simulink library "SimscapeCustomComponents_lib"  (R2025b)
settings: Solver=VariableStepAuto  StartTime=0.0  StopTime=10.0  RelTol=1e-3
undefined symbols (not defined in the file or in its folder): base, baseVdc, capacity, DiscIntNeverNeededParam, ee_sli_rtmsupport, filterInductance, freqeuncy, frequency, gcbh, gflInverter, gfmInverter, iMaxPU, Inertia, initialSOC, plantRating, solar, Ts, ups, Vac, windSystem, windTurbine
libraries: fl_lib x397, nesl_utility x171, eeGeneralControl x85, ee_lib x82, simulink x72, datacenter_lib x68, eeTransforms x38, slpidlib x24, buildingEnergy_lib x20, SimscapeFluids_lib x17, eeSinusoidalMeasurementV2 x8, eePwmGenerator x8
(part 19 of 24)

== system SimscapeCustomComponents_lib/Microgrid and Renewables/Control/BESS/Grid Forming Control/VoltageCurrentControl/Controller/Voltage control ==
  e : Inport
  resetBlackStart : Inport  Port=2
  Discrete-Time Integrator : DiscreteIntegrator  IntegratorMethod=Integration: Backward Euler  ExternalReset=level  SampleTime=voltControlTs  LimitOutput=on  UpperSaturationLimit=VdMaxCt  LowerSaturationLimit=VdMinCt  ICPrevOutput=DiscIntNeverNeededParam  ICPrevScaledInput=DiscIntNeverNeededParam
  Ki : Gain  Gain=VdIGain
  Kp : Gain  Gain=vdPGain
  Limit : Saturate  UpperLimit=VdMaxCt  LowerLimit=VdMinCt
  Scope : Scope  NumInputPorts=2
      settings: ActiveDisplayYMinimum=-2.29888  ActiveDisplayYMaximum=11.36654  DataLoggingVariableName=ScopeData7
  Scope1 : Scope
      settings: ActiveDisplayYMinimum=-0.22989  ActiveDisplayYMaximum=1.13665  DataLoggingVariableName=ScopeData8
  Sum7 : Sum  Inputs=|++
  u : Outport  VectorParamsAs1DForOutWhenUnconnected=off
  wires:
  Discrete-Time Integrator/1 -> Sum7/2, Scope/2
  Kp/1 -> Sum7/1, Scope/1
  Limit/1 -> u/1
  Ki/1 -> Discrete-Time Integrator/1
  Sum7/1 -> Limit/1
  e/1 -> Kp/1, Ki/1, Scope1/1
  resetBlackStart/1 -> Discrete-Time Integrator/2

== system SimscapeCustomComponents_lib/Microgrid and Renewables/Control/BESS/Grid Forming Control/VoltageCurrentControl/Controller/Voltage control1 ==
  e : Inport
  resetBlackStart : Inport  Port=2
  Discrete-Time Integrator : DiscreteIntegrator  IntegratorMethod=Integration: Backward Euler  ExternalReset=level  SampleTime=voltControlTs  LimitOutput=on  UpperSaturationLimit=VqMaxCt  LowerSaturationLimit=VqMinCt  ICPrevOutput=DiscIntNeverNeededParam  ICPrevScaledInput=DiscIntNeverNeededParam
  Ki : Gain  Gain=VqIGain
  Kp : Gain  Gain=VqPGain
  Limit : Saturate  UpperLimit=VqMaxCt  LowerLimit=VqMinCt
  Sum7 : Sum  Inputs=|++
  u : Outport  VectorParamsAs1DForOutWhenUnconnected=off
  wires:
  Discrete-Time Integrator/1 -> Sum7/2
  Sum7/1 -> Limit/1
  e/1 -> Ki/1, Kp/1
  Kp/1 -> Sum7/1
  Ki/1 -> Discrete-Time Integrator/1
  Limit/1 -> u/1
  resetBlackStart/1 -> Discrete-Time Integrator/2

== system SimscapeCustomComponents_lib/Microgrid and Renewables/Control/BESS/Grid Forming Control/VoltageCurrentControl/Controller/d-axis current control ==
  e : Inport
  resetBlackStart : Inport  Port=2
  Discrete-Time Integrator : DiscreteIntegrator  IntegratorMethod=Integration: Backward Euler  ExternalReset=level  SampleTime=currentControlTs  LimitOutput=on  UpperSaturationLimit=4  LowerSaturationLimit=-4  ICPrevOutput=DiscIntNeverNeededParam  ICPrevScaledInput=DiscIntNeverNeededParam
  Ki : Gain  Gain=IdIGain
  Kp : Gain  Gain=IdPGain
  Limit : Saturate  UpperLimit=4  LowerLimit=-4
  Sum7 : Sum  Inputs=|++
  u : Outport  VectorParamsAs1DForOutWhenUnconnected=off
  wires:
  Discrete-Time Integrator/1 -> Sum7/2
  Sum7/1 -> Limit/1
  e/1 -> Ki/1, Kp/1
  Kp/1 -> Sum7/1
  Limit/1 -> u/1
  Ki/1 -> Discrete-Time Integrator/1
  resetBlackStart/1 -> Discrete-Time Integrator/2

== system SimscapeCustomComponents_lib/Microgrid and Renewables/Control/BESS/Grid Forming Control/VoltageCurrentControl/Controller/q-axis current control ==
  e : Inport
  resetBlackStart : Inport  Port=2
  Discrete-Time Integrator : DiscreteIntegrator  IntegratorMethod=Integration: Backward Euler  ExternalReset=level  SampleTime=currentControlTs  LimitOutput=on  UpperSaturationLimit=3  LowerSaturationLimit=-3  ICPrevOutput=DiscIntNeverNeededParam  ICPrevScaledInput=DiscIntNeverNeededParam
  Ki : Gain  Gain=IqIGain
  Kp : Gain  Gain=IqPGain
  Limit : Saturate  UpperLimit=3  LowerLimit=-3
  Sum7 : Sum  Inputs=|++
  u : Outport  VectorParamsAs1DForOutWhenUnconnected=off
  wires:
  Ki/1 -> Discrete-Time Integrator/1
  Kp/1 -> Sum7/1
  e/1 -> Kp/1, Ki/1
  Sum7/1 -> Limit/1
  Limit/1 -> u/1
  Discrete-Time Integrator/1 -> Sum7/2
  resetBlackStart/1 -> Discrete-Time Integrator/2

== system SimscapeCustomComponents_lib/Microgrid and Renewables/Control/Renewables/Power Reference Controller/Power Reference Controller/Reference Current/Current limits ==
  Imax : Inport
  iqref : Inport  Port=2
  idref : Inport  Port=3
  Constant8 : Constant  Value=0
  Constant9 : Constant  Value=0
  Scope : Scope
      settings: ActiveDisplayYMinimum=-0.15  ActiveDisplayYMaximum=1.35  DataLoggingVariableName=ScopeData3
  Scope1 : Scope
      settings: ActiveDisplayYMinimum=-0.08298  ActiveDisplayYMaximum=0.74678  DataLoggingVariableName=ScopeData4
  Sqrt : Sqrt
  Sqrt1 : Sqrt
  Square{1..4} (4 alike) : Math  Operator=square
  Step2 : Step  Time=0.01  SampleTime=Ts
  Step3 : Step  Time=0.01  SampleTime=Ts
  Sum6 : Sum  Inputs=|+-
  Sum9 : Sum  Inputs=|+-
  Switch1 : Switch  Threshold=.01  SaturateOnIntegerOverflow=off  InputSameDT=off
  Switch2 : Switch  Threshold=.01  SaturateOnIntegerOverflow=off  InputSameDT=off
  iubq : Outport
  iubd : Outport  Port=2
  wires:
  Sum9/1 -> Switch2/1
  Step3/1 -> Switch2/2
  Step2/1 -> Switch1/2
  Switch2/1 -> Sqrt1/1
  Square1/1 -> Sum6/1
  Switch1/1 -> Sqrt/1
  iqref/1 -> Square2/1
  Square3/1 -> Sum9/1
  Sum6/1 -> Switch1/1
  Square2/1 -> Sum6/2
  Constant8/1 -> Switch1/3
  Square4/1 -> Sum9/2
  Constant9/1 -> Switch2/3
  Sqrt/1 -> Scope/1, iubd/1
  Imax/1 -> Square3/1, Square1/1
  Sqrt1/1 -> Scope1/1, iubq/1
  idref/1 -> Square4/1

== system SimscapeCustomComponents_lib/Microgrid and Renewables/Control/Renewables/Power Reference Controller/Power Reference Controller/Reference Current/Refernce id generation ==
  V_mag : Inport
  ubid : Inport  Port=2
  PRef : Inport  Port=3
  Divide : Product  Inputs=/*
  Gain6 : Gain  Gain=-1
  P/Q Priority : Switch  Criteria=u2 ~= 0  SaturateOnIntegerOverflow=off  InputSameDT=off
  Priority Mode : Constant  Value=P-2
  Saturation Dynamic2 : simulink/Discontinuities/Saturation Dynamic  OutMin=[]  OutMax=[]  OutDataTypeStr=Inherit: Same as second input  OutDataType=fixdt(1, 16)  OutScaling=2^-10  DoSatur=off
  Saturation1 : Saturate  UpperLimit=Imax  LowerLimit=-Imax
  Scope : Scope
      settings: ActiveDisplayYMinimum=0.99583  ActiveDisplayYMaximum=1.02853
  Scope1 : Scope
      settings: ActiveDisplayYMinimum=-0.12499  ActiveDisplayYMaximum=1.12489  DataLoggingVariableName=ScopeData2
  ubid1 : InportShadow  Port=2
  id_ref : Outport
  wires:
  PRef/1 -> Divide/2
  ubid/1 -> Saturation Dynamic2/1
  Gain6/1 -> Saturation Dynamic2/3
  Saturation Dynamic2/1 -> Scope1/1, P/Q Priority/3
  Priority Mode/1 -> P/Q Priority/2
  Saturation1/1 -> P/Q Priority/1
  ubid1/1 -> Gain6/1
  P/Q Priority/1 -> Scope/1, id_ref/1
  V_mag/1 -> Divide/1
  Divide/1 -> Saturation Dynamic2/2, Saturation1/1

== system SimscapeCustomComponents_lib/Microgrid and Renewables/Control/Renewables/Power Reference Controller/Power Reference Controller/Reference Current/Refernce iq generation ==
  ubiq : Inport
  V_mag : Inport  Port=2
  LVRT_iq : Inport  Port=3
  Q_ref : Inport  Port=4
  Divide1 : Product  Inputs=*/
  Gain : Gain  Gain=-1
  Gain1 : Gain  Gain=-1
  Gain7 : Gain  Gain=-1
  LVRT Priority : Switch  Threshold=.9  SaturateOnIntegerOverflow=off  InputSameDT=off
  P/Q Priority : Switch  Criteria=u2 ~= 0  SaturateOnIntegerOverflow=off  InputSameDT=off
  Priority Mode : Constant  Value=P-2
  Saturation Dynamic : simulink/Discontinuities/Saturation Dynamic  OutMin=[]  OutMax=[]  OutDataTypeStr=Inherit: Same as second input  OutDataType=fixdt(1, 16)  OutScaling=2^-10  DoSatur=off
  Saturation2 : Saturate  UpperLimit=1  LowerLimit=-1
  Saturation3 : Saturate  UpperLimit=Imax  LowerLimit=-Imax
  Scope : Scope  NumInputPorts=3
      settings: ActiveDisplayYMinimum=-0.025  ActiveDisplayYMaximum=0.22499  DataLoggingVariableName=ScopeData10
  ubiq1 : InportShadow
  iq_ref : Outport
  wires:
  LVRT Priority/1 -> Gain/1
  P/Q Priority/1 -> LVRT Priority/1, Scope/1
  Gain1/1 -> LVRT Priority/3
  ubiq/1 -> Saturation Dynamic/1
  Saturation2/1 -> Gain1/1
  Saturation3/1 -> P/Q Priority/3
  Priority Mode/1 -> P/Q Priority/2
  Divide1/1 -> Saturation3/1, Saturation Dynamic/2
  Saturation Dynamic/1 -> P/Q Priority/1
  Gain7/1 -> Saturation Dynamic/3
  LVRT_iq/1 -> Saturation2/1
  ubiq1/1 -> Gain7/1
  Q_ref/1 -> Divide1/1
  V_mag/1 -> LVRT Priority/2, Divide1/2
  Gain/1 -> iq_ref/1

== system SimscapeCustomComponents_lib/Microgrid and Renewables/Control/Renewables/Solar PV Controller/DC voltage controller & current reference/If Action Subsystem/Subsystem ==
  V mag : Inport
  iq ub : Inport  Port=2
  Q ref : Inport  Port=3
  Constant : Constant  Value=1e-3
  Data Type Conversion Inherited : simulink/Signal Attributes/Data Type Conversion Inherited  ConvertRealWorld=Real World Value  DoSatur=off
  Divide2 : Product  Inputs=*/
  Gain3 : Gain  Gain=-1
  Saturation Dynamic2 : simulink/Discontinuities/Saturation Dynamic  OutMin=[]  OutMax=[]  OutDataTypeStr=Inherit: Same as second input  OutDataType=fixdt(1, 16)  OutScaling=2^-10  DoSatur=off
  Switch : Switch  Criteria=u2 ~= 0  SaturateOnIntegerOverflow=off  InputSameDT=off
  iq ub1 : InportShadow  Port=2
  iqref : Outport
  wires:
  iq ub1/1 -> Gain3/1
  Divide2/1 -> Saturation Dynamic2/2
  Q ref/1 -> Divide2/1
  Gain3/1 -> Saturation Dynamic2/3
  iq ub/1 -> Saturation Dynamic2/1
  Saturation Dynamic2/1 -> iqref/1
  V mag/1 -> Data Type Conversion Inherited/1, Switch/2, Switch/1
  Switch/1 -> Divide2/2
  Constant/1 -> Data Type Conversion Inherited/2
  Data Type Conversion Inherited/1 -> Switch/3

== system SimscapeCustomComponents_lib/Microgrid and Renewables/Control/Renewables/Solar PV Controller/DC voltage controller & current reference/If Action Subsystem/Subsystem1 ==
  Vmag : Inport
  P pv : Inport  Port=2
  vdc : Inport  Port=3
  vdc ref : Inport  Port=4
  id ub : Inport  Port=5
  Constant : Constant  Value=1e-3
  Constant4 : Constant  Value=0
  Data Type Conversion Inherited : simulink/Signal Attributes/Data Type Conversion Inherited  ConvertRealWorld=Real World Value  DoSatur=off
  Divide : Product  Inputs=/*
  Gain4 : Gain  Gain=1/(mVAbase)
  Saturation Dynamic1 : simulink/Discontinuities/Saturation Dynamic  OutMin=[]  OutMax=[]  OutDataTypeStr=Inherit: Same as second input  OutDataType=fixdt(1, 16)  OutScaling=2^-10  DoSatur=off
  Scope : Scope  NumInputPorts=2
      settings: ActiveDisplayYMinimum=-55957.97767  ActiveDisplayYMaximum=503630.2665
  Sum : Sum  Inputs=|++
  Switch : Switch  Criteria=u2 ~= 0  SaturateOnIntegerOverflow=off  InputSameDT=off
  V_dc_Controller1 : Subsystem
  idref : Outport
  wires:
  Constant4/1 -> Saturation Dynamic1/3
  P pv/1 -> Gain4/1
  V_dc_Controller1/1(Out1) -> Sum/2
  Sum/1 -> Saturation Dynamic1/2
  vdc ref/1 -> V_dc_Controller1/2(vdc ref), Scope/2
  id ub/1 -> Saturation Dynamic1/1
  Gain4/1 -> Divide/2
  Divide/1 -> Sum/1
  Saturation Dynamic1/1 -> idref/1
  vdc/1 -> V_dc_Controller1/1(vdc), Scope/1
  Vmag/1 -> Data Type Conversion Inherited/1, Switch/2, Switch/1
  Switch/1 -> Divide/1
  Constant/1 -> Data Type Conversion Inherited/2
  Data Type Conversion Inherited/1 -> Switch/3

== system SimscapeCustomComponents_lib/Microgrid and Renewables/Control/Renewables/Solar PV Controller/DC voltage controller & current reference/Subsystem1/V_dc_Controller1 ==
  vdc : Inport
  vdc ref : Inport  Port=2
  Gain : Gain  Gain=1/VdcBase
  PID Controller : slpidlib/PID Controller  Controller=PID  Form=Parallel  TimeDomain=Discrete-time  UseExternalTs=off  SampleTime=-1  IntegratorMethod=Forward Euler  FilterMethod=Forward Euler  ControllerParametersSource=internal  P=Kpv  I=Kiv  UseKiTs=off  D=Kdv  UseExternalDerivativeSource=off  N=100  UseFilter=on  TunerSelectOption=Transfer Function Based (PID Tuner App)  ZeroCross=off  InitialConditionSource=internal  InitialConditionForIntegrator=0  InitialConditionForFilter=0  DifferentiatorICPrevScaledInput=0  ExternalReset=none  TrackingMode=off  Kt=1  LimitOutput=off  SatLimitsSource=internal  UpperSaturationLimit=iMax  LowerSaturationLimit=0  LinearizeAsGain=on  AntiWindupMode=clamping  Kb=1  LimitIntegrator=off  UpperIntegratorSaturationLimit=inf  LowerIntegratorSaturationLimit=-inf  POutMin=[]  POutMax=[]  IOutMin=[]  IOutMax=[]  DOutMin=[]  DOutMax=[]  NOutMin=[]  NOutMax=[]  SumOutMin=[]  SumOutMax=[]  SaturationOutMin=[]  SaturationOutMax=[]  PParamMin=[]  PParamMax=[]  IParamMin=[]  IParamMax=[]  DParamMin=[]  DParamMax=[]  NParamMin=[]  NParamMax=[]  KbParamMin=[]  KbParamMax=[]  KtParamMin=[]  KtParamMax=[]  KbOutMin=[]  KbOutMax=[]  KtOutMin=[]  KtOutMax=[]  IntegratorOutMin=[]  IntegratorOutMax=[]  FilterOutMin=[]  FilterOutMax=[]  SumI1OutMin=[]  SumI1OutMax=[]  SumI2OutMin=[]  SumI2OutMax=[]  SumI3OutMin=[]  SumI3OutMax=[]  SumI4OutMin=[]  SumI4OutMax=[]  SumDOutMin=[]  SumDOutMax=[]  DifferentiatorOutMin=[]  DifferentiatorOutMax=[]  FilterDiffOutCoefMin=[]  FilterDiffOutCoefMax=[]  ReciprocalOutMin=[]  ReciprocalOutMax=[]  SumDenOutMin=[]  SumDenOutMax=[]  SumNumOutMin=[]  SumNumOutMax=[]  DivideOutMin=[]  DivideOutMax=[]  UdiffTsProdOutMin=[]  UdiffTsProdOutMax=[]  NTsProdOutMin=[]  NTsProdOutMax=[]  UintegralTsProdOutMin=[]  UintegralTsProdOutMax=[]  UngainTsProdOutMin=[]  UngainTsProdOutMax=[]  ClampingZeroOutDataTypeStr=Inherit: Inherit via back propagation  ClampingZeroOutMin=[]  ClampingZeroOutMax=[]  FilterDenConstantOutDataTypeStr=Inherit: Inherit via back propagation  FilterDenConstantOutMin=[]  FilterDenConstantOutMax=[]  PCopyOutDataTypeStr=Inherit: Inherit via back propagation  PCopyOutMin=[]  PCopyOutMax=[]  NCopyOutDataTypeStr=Inherit: Inherit via back propagation  NCopyOutMin=[]  NCopyOutMax=[]  IntegratorContinuousStateAttributes=''  IntegratorStateMustResolveToSignalObject=off  IntegratorRTWStateStorageClass=Auto  FilterContinuousStateAttributes=''  FilterStateMustResolveToSignalObject=off  FilterRTWStateStorageClass=Auto  ParallelPVariant=InternalParameters  IdealPVariant=Disabled  IVariant=InternalParameters  DVariant=InternalParameters  IntegratorVariant=Discrete  SatVariant=Disabled  AWVariant=Passthrough  PCopyVariant=Disabled  TRVariant=Disabled  FdbkBlocksVariant=Forward  IdealPFdbkVariant=Disabled  SatFdbkVariant=Disabled  DerivativeFilterVariant=ForwardEulerFilter  NVariant=InternalParameters  NCopyVariant=Disabled  FilterICVariant=InternalICsFilter  IntegratorICVariant=InternalICs  ExternalResetVariant=Disabled  TRSumVariant=Passthrough  SumFdbkVariant=Disabled  SumVariant=Sum_PID  TsampFilterVariant=InternalTs  TsampNgainVariant=Passthrough  TsampIntegralVariant=Disabled_SignalSpec  ExternalSaturationOutDataTypeStr=Inherit: Same as second input  DerivativeSourceVariant=ErrorSignal  PreIntVariant=InternalPreInt
  Sum : Sum  Inputs=|+-
  Out1 : Outport
  wires:
  vdc/1 -> Sum/1
  vdc ref/1 -> Sum/2
  PID Controller/1 -> Out1/1
  Gain/1 -> PID Controller/1
  Sum/1 -> Gain/1

== system SimscapeCustomComponents_lib/Microgrid and Renewables/Control/Renewables/Wind Controller/Machine Converter Control/Power Controller/Derating Control ==
  Enable : EnablePort  StatesWhenEnabling=reset
  Constant : Constant  Value=windTurbine.turbineRatedPower
  MW to W : Gain  Gain=1e6
  activePowerDemand : Outport
  wires:
  MW to W/1 -> activePowerDemand/1
  Constant/1 -> MW to W/1

== system SimscapeCustomComponents_lib/Microgrid and Renewables/Control/Renewables/Wind Controller/Machine Converter Control/Power Controller/Limiter Function Power Demand ==
  activePowerDemandMPPT : Inport
  activePowerDemandDerating : Inport  Port=2
  Merge : Merge
  activePowerDemand : Outport
  wires:
  activePowerDemandMPPT/1 -> Merge/1
  activePowerDemandDerating/1 -> Merge/2
  Merge/1 -> activePowerDemand/1

== system SimscapeCustomComponents_lib/Microgrid and Renewables/Control/Renewables/Wind Controller/Machine Converter Control/Power Controller/MPPT Control ==
  windSpeed : Inport
  Enable : EnablePort  StatesWhenEnabling=reset
  MW to W : Gain  Gain=1e6
  mpptActivePowerDemand : Lookup_n-D  NumberOfTableDimensions=1  BreakpointsForDimension1=mpptWindSpeed  Table=mpptPower  InternalRulePriority=Speed  RndMeth=Simplest
  activePowerDemand : Outport
  wires:
  mpptActivePowerDemand/1 -> MW to W/1
  windSpeed/1 -> mpptActivePowerDemand/1
  MW to W/1 -> activePowerDemand/1

== system SimscapeCustomComponents_lib/Microgrid and Renewables/Control/Renewables/Wind Controller/Wind Grid-side Converter Controller/Current_controller/PI ==
  Input : Inport
  Discrete-Time Integrator : DiscreteIntegrator  gainval=Kdii_g  SampleTime=Ts  ICPrevOutput=DiscIntNeverNeededParam  ICPrevScaledInput=DiscIntNeverNeededParam
  Gain1 : Gain  Gain=Kdpi_g
  Sum1 : Sum  Inputs=|++
  Unit Delay : UnitDelay  SampleTime=Ts
  Out2 : Outport
  wires:
  Discrete-Time Integrator/1 -> Sum1/1
  Sum1/1 -> Out2/1
  Unit Delay/1 -> Sum1/2
  Gain1/1 -> Unit Delay/1
  Input/1 -> Gain1/1, Discrete-Time Integrator/1

== system SimscapeCustomComponents_lib/Microgrid and Renewables/Control/Renewables/Wind Controller/Wind Grid-side Converter Controller/Current_controller/PI1 ==
  Input : Inport
  Discrete-Time Integrator : DiscreteIntegrator  gainval=Kqii_g  SampleTime=Ts  ICPrevOutput=DiscIntNeverNeededParam  ICPrevScaledInput=DiscIntNeverNeededParam
  Gain1 : Gain  Gain=Kqpi_g
  Sum1 : Sum  Inputs=|++
  Unit Delay : UnitDelay  SampleTime=Ts
  Out2 : Outport
  wires:
  Discrete-Time Integrator/1 -> Sum1/1
  Sum1/1 -> Out2/1
  Unit Delay/1 -> Sum1/2
  Gain1/1 -> Unit Delay/1
  Input/1 -> Gain1/1, Discrete-Time Integrator/1

== system SimscapeCustomComponents_lib/Microgrid and Renewables/Control/Renewables/Wind Controller/Wind Grid-side Converter Controller/DC voltage controller & current reference/Current limits ==
  Imax : Inport
  iqref : Inport  Port=2
  idref : Inport  Port=3
  Constant8 : Constant  Value=0
  Constant9 : Constant  Value=0
  Sqrt : Sqrt
  Sqrt1 : Sqrt
  Square{1..4} (4 alike) : Math  Operator=square
  Step2 : Step  Time=0.01  SampleTime=Ts
  Step3 : Step  Time=0.01  SampleTime=Ts
  Sum6 : Sum  Inputs=|+-
  Sum9 : Sum  Inputs=|+-
  Switch1 : Switch  Threshold=.01  SaturateOnIntegerOverflow=off  InputSameDT=off
  Switch2 : Switch  Threshold=.01  SaturateOnIntegerOverflow=off  InputSameDT=off
  iubq : Outport
  iubd : Outport  Port=2
  wires:
  Sum9/1 -> Switch2/1
  Step3/1 -> Switch2/2
  Step2/1 -> Switch1/2
  Switch2/1 -> Sqrt1/1
  Square1/1 -> Sum6/1
  Switch1/1 -> Sqrt/1
  iqref/1 -> Square2/1
  Square3/1 -> Sum9/1
  Sum6/1 -> Switch1/1
  Square2/1 -> Sum6/2
  Constant8/1 -> Switch1/3
  Square4/1 -> Sum9/2
  Constant9/1 -> Switch2/3
  Sqrt/1 -> iubd/1
  Imax/1 -> Square3/1, Square1/1
  Sqrt1/1 -> iubq/1
  idref/1 -> Square4/1

== system SimscapeCustomComponents_lib/Microgrid and Renewables/Control/Renewables/Wind Controller/Wind Grid-side Converter Controller/DC voltage controller & current reference/Subsystem ==
  V_mag : Inport
  iq_ub : Inport  Port=2
  lvrt.iq : Inport  Port=3
  Q_ref : Inport  Port=4
  Divide2 : Product  Inputs=*/
  Gain3 : Gain  Gain=-1
  Saturation Dynamic2 : simulink/Discontinuities/Saturation Dynamic  OutMin=[]  OutMax=[]  OutDataTypeStr=Inherit: Same as second input  OutDataType=fixdt(1, 16)  OutScaling=2^-10  DoSatur=off
  Switch6 : Switch  Threshold=.9  SaturateOnIntegerOverflow=off  InputSameDT=off
  iq_ub1 : InportShadow  Port=2
  Out1 : Outport
  wires:
  V_mag/1 -> Switch6/2, Divide2/2
  iq_ub1/1 -> Gain3/1
  Divide2/1 -> Saturation Dynamic2/2
  Q_ref/1 -> Divide2/1
  Gain3/1 -> Saturation Dynamic2/3
  iq_ub/1 -> Saturation Dynamic2/1
  Saturation Dynamic2/1 -> Switch6/1
  Switch6/1 -> Out1/1
  lvrt.iq/1 -> Switch6/3

== system SimscapeCustomComponents_lib/Microgrid and Renewables/Control/Renewables/Wind Controller/Wind Grid-side Converter Controller/DC voltage controller & current reference/Subsystem1 ==
  Wind_Mpp_vdc : Inport
  Wind_vdc : Inport  Port=2
  id_ub : Inport  Port=3
  Constant4 : Constant  Value=0
  Saturation Dynamic1 : simulink/Discontinuities/Saturation Dynamic  OutMin=[]  OutMax=[]  OutDataTypeStr=Inherit: Same as second input  OutDataType=fixdt(1, 16)  OutScaling=2^-10  DoSatur=off
  V_dc_Controller1 : Subsystem
  Out1 : Outport
  wires:
  Constant4/1 -> Saturation Dynamic1/3
  V_dc_Controller1/1(Out1) -> Saturation Dynamic1/2
  Wind_vdc/1 -> V_dc_Controller1/2(In2)
  id_ub/1 -> Saturation Dynamic1/1
  Saturation Dynamic1/1 -> Out1/1
  Wind_Mpp_vdc/1 -> V_dc_Controller1/1(Wind_plant1)

== system SimscapeCustomComponents_lib/Microgrid and Renewables/Sources/Solar Plant Integrated/Detailed/PV Plant & Controller/Controller/MPPT ==
  Qref : Inport
  ipv (A) : Inport  Port=2
  vdc (V) : Inport  Port=3
  Vabc : Inport  Port=4
  Iabc : Inport  Port=5
  Action Port : ActionPort
  Solar PV Controller : Subsystem  LoadFcn=ee_sli_rtmsupport( 'loadfcn', gcbh );  mask(Solar PV Controller (Three-Phase)){L=filterInductance, frequency=frequency, iMax=iMaxPU, zBase=Vac^2/(plantRating*1000), mVAbase=plantRating*1000, VdcBase=baseVoltageDC, sampleTime=-1, Choice=Perturb and observe (P&O), Vdc=1100, delV=3, tSettling=1e-3, Kppll=1e-4, Kipll=0.02, initialPhase=0, Kpv=0.1, Kiv=1, Kdv=0, Kpicd=0.01, Kiicd=0.1, Kdicd=0, Kpicq=0.01, Kiicq=0.1, Kdicq=0}
      mask prompts: L "physmod:ee:library:comments:control:eeRenewablesControl:ACFilterInductanceH_MP"; frequency "physmod:ee:library:comments:control:eeRenewablesControl:SystemFrequencyHz_MP"; iMax "physmod:ee:library:comments:control:eeRenewablesControl:InverterCurrentLimitpu_MP"; zBase "physmod:ee:library:comments:control:eeRenewablesControl:BaseImpedanceACSideOhm_MP"; mVAbase "physmod:ee:library:comments:control:eeRenewablesControl:BaseMVA_MP"; VdcBase "physmod:ee:library:comments:control:eeRenewablesControl:DCBusBaseVoltageV_MP"; sampleTime "physmod:ee:library:comments:control:eeRenewablesControl:SampleTime1ForInherited_MP"; Choice "physmod:ee:library:comments:control:eeRenewablesControl:Algorithm_MP"; Vdc "physmod:ee:library:comments:control:eeRenewablesControl:InitialVoltageForMPPTV_MP"; delV "physmod:ee:library:comments:control:eeRenewablesControl:VoltageStepOfMPPTV_MP"; tSettling "physmod:ee:library:comments:control:eeRenewablesControl:SettlingTimeOfMPPTs_MP"; Kppll "physmod:ee:library:comments:control:eeRenewablesControl:ProportionalGain_MP"; Kipll "physmod:ee:library:comments:control:eeRenewablesControl:IntegralGain_MP"; initialPhase "physmod:ee:library:comments:control:eeRenewablesControl:InitialPhaseAngle_MP"; Kpv "physmod:ee:library:comments:control:eeRenewablesControl:ProportionalGain_MP"; Kiv "physmod:ee:library:comments:control:eeRenewablesControl:IntegralGain_MP"; Kdv "physmod:ee:library:comments:control:eeRenewablesControl:DerivativeGain_MP"; Kpicd "physmod:ee:library:comments:control:eeRenewablesControl:DaxisProportionalGain_MP"; Kiicd "physmod:ee:library:comments:control:eeRenewablesControl:DaxisIntegralGain_MP"; Kdicd "physmod:ee:library:comments:control:eeRenewablesControl:DaxisDerivativeGain_MP"; Kpicq "physmod:ee:library:comments:control:eeRenewablesControl:QaxisProportionalGain_MP"; Kiicq "physmod:ee:library:comments:control:eeRenewablesControl:QaxisIntegralGain_MP"; Kdicq "physmod:ee:library:comments:control:eeRenewablesControl:QaxisDerivativeGain_MP"
      mask help: physmod:ee:library:comments:control:eeRenewablesControl:PVGridFollowingController_MD
      mask init: same as SimscapeCustomComponents_lib/Microgrid and Renewables/Control/Renewables/Solar PV Controller
      settings: CopyFcn=ee_sli_rtmsupport( 'copyfcn', gcbh );  DeleteFcn=ee_sli_rtmsupport( 'deletefcn', gcbh );  ModelCloseFcn=ee_sli_rtmsupport( 'modelclosefcn', gcbh );  PostSaveFcn=ee_sli_rtmsupport( 'postsavefcn', gcbh );  PreCopyFcn=ee_sli_rtmsupport( 'precopyfcn', gcbh );  OpenFcn=ee_sli_rtmsupport( 'openfcn', gcbh );  CloseFcn=ee_sli_rtmsupport( 'closefcn', gcbh );  PreDeleteFcn=ee_sli_rtmsupport( 'predeletefcn', gcbh );
      mask Help: web(nesl_help(gcbh))
      mask TypeOptions sampleTime: Current_controller/SystemSampleTime | DC voltage controller & current reference/SystemSampleTime
      mask TypeOptions Choice: Variant Subsystem/LabelModeActiveChoice
      mask DialogControl Container4 Prompt: physmod:ee:library:comments:control:eeRenewablesControl:General_Tab
      mask DialogControl L Prompt: AC filter inductance (H)
      mask DialogControl frequency Prompt: System frequency (Hz)
      mask DialogControl iMax Prompt: Inverter current limit (pu)
      mask DialogControl zBase Prompt: Base impedance on AC side (Ohm)
      mask DialogControl mVAbase Prompt: Base power on AC side (V*A)
      mask DialogControl VdcBase Prompt: DC bus base voltage (V)
      mask DialogControl sampleTime Prompt: Sample time (-1 for inherited)
      mask DialogControl Container5 Prompt: physmod:ee:library:comments:control:eeRenewablesControl:MPPT_Tab
      mask DialogControl Choice Prompt: Algorithm
      mask DialogControl Vdc Prompt: Initial voltage for MPPT (V)
      mask DialogControl delV Prompt: Voltage step of MPPT (V)
      mask DialogControl tSettling Prompt: Settling time of MPPT (s)
      mask DialogControl Container6 Prompt: physmod:ee:library:comments:control:eeRenewablesControl:PLL_Tab
      mask DialogControl Kppll Prompt: Proportional gain
      mask DialogControl Kipll Prompt: Integral gain
      mask DialogControl initialPhase Prompt: Initial phase angle (deg)
      mask DialogControl Container7 Prompt: physmod:ee:library:comments:control:eeRenewablesControl:VoltageController_Tab
      mask DialogControl Kpv Prompt: Proportional gain
      mask DialogControl Kiv Prompt: Integral gain
      mask DialogControl Kdv Prompt: Derivative gain
      mask DialogControl Container8 Prompt: physmod:ee:library:comments:control:eeRenewablesControl:CurrentController_Tab
      mask DialogControl Kpicd Prompt: D-axis proportional gain
      mask DialogControl Kiicd Prompt: D-axis integral gain
      mask DialogControl Kdicd Prompt: D-axis derivative gain
      mask DialogControl Kpicq Prompt: Q-axis proportional gain
      mask DialogControl Kiicq Prompt: Q-axis integral gain
      mask DialogControl Kdicq Prompt: Q-axis derivative gain
      mask Display: ee.mask.drawPVcontroller;
  mabc : Outport
  wires:
  Solar PV Controller/1(vabcRef (pu)) -> mabc/1
  Qref/1 -> Solar PV Controller/1(Qref (pu))
  vdc (V)/1 -> Solar PV Controller/3(vdc (V))
  Vabc/1 -> Solar PV Controller/4(vabc (pu))
  Iabc/1 -> Solar PV Controller/5(iabc (pu))
  ipv (A)/1 -> Solar PV Controller/2(ipv (A))

== system SimscapeCustomComponents_lib/Microgrid and Renewables/Sources/Solar Plant Integrated/Detailed/PV Plant & Controller/Controller/Power Reference ==
  Iabc : Inport
  Vabc : Inport  Port=2
  PRef : Inport  Port=3
  QRef : Inport  Port=4
  Action Port : ActionPort
  Power Reference Controller : Subsystem  mask(Power Reference Controller){frequency=frequency, P=Real power, MVA=plantRating, zbase=Vac^2/plantRating, L=filterInductance, Imax=iMaxPU, Td=1e-3, Kpic=1.5, Kiic=10, Kd=0, kpPLL=40, kiPLL=1000, kdPLL=0}
      mask prompts: frequency "Frequency (Hz)"; P "Priority mode"; MVA "Base Power (V*A)"; zbase "Base Impedance (Ohm)"; L "Filter Inductance (H)"; Imax "Inverter current limit (pu)"; Td "Sensor time delay (s)"; Kpic "Proportional gain"; Kiic "Integral gain"; Kd "Derevative gain"; kpPLL "Proportional gain"; kiPLL "Integral gain"; kdPLL "Derevative gain"
      mask help: This block receives active and reactive power references for the converter based on system requirements or higher-level control commands. It ensures that the converter operates according to desired power setpoints, supporting grid services such as frequency regulation, voltage support, and power dispatch
      settings: CopyFcn=set_param(gcbh,'LinkStatus','none');
      mask TypeOptions P: Real power  | Reactive power
      mask DialogControl Container4 Prompt: General
      mask DialogControl Container5 Prompt: Current Controller
      mask DialogControl Container5_copy Prompt: PLL
  mabc : Outport
  wires:
  Iabc/1 -> Power Reference Controller/1(Iabc)
  Vabc/1 -> Power Reference Controller/2(Vabc)
  Power Reference Controller/1(mabc) -> mabc/1
  PRef/1 -> Power Reference Controller/3(Pref)
  QRef/1 -> Power Reference Controller/4(Qref)

== system SimscapeCustomComponents_lib/Microgrid and Renewables/Sources/Solar Plant Integrated/Detailed/PV Plant & Controller/PV Plant/Converter ==
  mabc : Inport
  Average : Subsystem  VariantControl=Average
  Switching : Subsystem  VariantControl=Switching
  + : PMIOPort  Side=Left
  - : PMIOPort  Port=2  Side=Left
  ~ : PMIOPort  Port=3  Side=Right

== system SimscapeCustomComponents_lib/Microgrid and Renewables/Sources/Solar Plant Integrated/Detailed/PV Plant & Controller/Sensor Dynamics/Current Measurement ==
  u : Inport
  Lead-Lag (Discrete or Continuous) : eeGeneralControl/Lead-Lag (Discrete or Continuous)  T1=0  T2=PV.controllerTSensor  B=inf  A=-inf  init_option=Inherited from block input  x0=0  Ts=Ts
  V : Outport
  wires:
  Lead-Lag (Discrete or Continuous)/1 -> V/1
  u/1 -> Lead-Lag (Discrete or Continuous)/1

== system SimscapeCustomComponents_lib/Microgrid and Renewables/Sources/Solar Plant Integrated/Detailed/PV Plant & Controller/Sensor Dynamics/Voltage Measurement ==
  u : Inport
  Lead-Lag (Discrete or Continuous) : eeGeneralControl/Lead-Lag (Discrete or Continuous)  T1=0  T2=PV.controllerTSensor  B=inf  A=-inf  init_option=Inherited from block input  x0=0  Ts=Ts
  I : Outport
  wires:
  Lead-Lag (Discrete or Continuous)/1 -> I/1
  u/1 -> Lead-Lag (Discrete or Continuous)/1

== system SimscapeCustomComponents_lib/Microgrid and Renewables/Sources/Wind Plant/Back-to-Back Converters/Switching/Grid Side Converter/Pulse Generation1 ==
  G : Inport
  Constant : Constant  Value=5
  Subtract : Sum  Inputs=-+
  G1 : Outport  VectorParamsAs1DForOutWhenUnconnected=off
  G2 : Outport  Port=2  VectorParamsAs1DForOutWhenUnconnected=off
  wires:
  Subtract/1 -> G2/1
  Constant/1 -> Subtract/2
  G/1 -> G1/1, Subtract/1

== system SimscapeCustomComponents_lib/Microgrid and Renewables/Sources/Wind Plant/Back-to-Back Converters/Switching/Machine Side Converter/Pulse Generation ==
  G : Inport
  Constant : Constant  Value=5
  Subtract : Sum  Inputs=-+
  G1 : Outport  VectorParamsAs1DForOutWhenUnconnected=off
  G2 : Outport  Port=2  VectorParamsAs1DForOutWhenUnconnected=off
  wires:
  Subtract/1 -> G2/1
  Constant/1 -> Subtract/2
  G/1 -> G1/1, Subtract/1

== system SimscapeCustomComponents_lib/Microgrid and Renewables/Sources/Wind Plant Integrated/Detailed/PLL/PLL & Measurements1/Subsystem ==
  Vabc : Inport
  Iabc : Inport  Port=2
  Demux : Demux  Outputs=3
  Demux1 : Demux  Outputs=3
  Park Transform : eeTransforms/Park Transform  AxisAlignment=Q-axis  PowerInvariant=off
  Park Transform1 : eeTransforms/Park Transform  AxisAlignment=Q-axis  PowerInvariant=off
  Scope : Scope  NumInputPorts=2
      settings: ActiveDisplayYMinimum=0.95416  ActiveDisplayYMaximum=1.02793  DataLoggingVariableName=ScopeData5
  "Sinusoidal Measurement (PLL, Three-Phase)" : eeSinusoidalMeasurementV2/Sinusoidal Measurement (PLL, Three-Phase)  InputFilter=on  InputNormalization=off  Kp_LF=100  Ki_LF=2000  F0=50  Theta0=0  Ts=Ts
  Terminator : Terminator
  Terminator1 : Terminator
  mag : Outport
  freq : Outport  Port=2
  angle : Outport  Port=3
  Vd : Outport  Port=4
  Vq : Outport  Port=5
  Id1 : Outport  Port=6
  Iq1 : Outport  Port=7
  wires:
  Iabc/1 -> Park Transform1/1
  Demux1/3 -> Terminator1/1
  Demux1/2 -> Iq1/1
  Demux1/1 -> Id1/1
  Park Transform1/1 -> Demux1/1
  "Sinusoidal Measurement (PLL, Three-Phase)"/3 -> mag/1
  "Sinusoidal Measurement (PLL, Three-Phase)"/1 -> freq/1
  "Sinusoidal Measurement (PLL, Three-Phase)"/2 -> Park Transform/2, Park Transform1/2, angle/1
  Demux/2 -> Vq/1, Scope/2
  Demux/1 -> Vd/1, Scope/1
  Park Transform/1 -> Demux/1
  Vabc/1 -> "Sinusoidal Measurement (PLL, Three-Phase)"/1, Park Transform/1
  Demux/3 -> Terminator/1

== system SimscapeCustomComponents_lib/Microgrid and Renewables/Sources/Wind Plant Integrated/Detailed/Wind Turbine and Converters/Wind Controller/Machine Converter Control ==
  iabc_sens : Inport
  w_sens : Inport  Port=2
  a_sens : Inport  Port=3
  vdc_sens : Inport  Port=4
  Wind speed : Inport  Port=5
  LVRT : Inport  Port=6
  Constant : Constant  Value=0  SampleTime=-1
  Constant1 : Constant  Value=(2/3)
  Constant2 : Constant  Value=psim
  Constant3 : Constant  Value=0
  Constant4 : Constant  Value=2*pi*20
  Constant5 : Constant  Value=1000  VectorParams1D=off  SampleTime=-1
  Constant6 : Constant  Value=0
  Divide : Product  Inputs=*//
  Divide1 : Product  Inputs=*/
  Gain : Gain  Gain=p
  Gain1 : Gain  Gain=2
  Gain2 : Gain  Gain=-1
  Inverse Park Transform : eeTransforms/Inverse Park Transform  AxisAlignment=Q-axis  PowerInvariant=off
  Measurements : Subsystem
  Mux : Mux  Inputs=2
  Mux1 : Mux  Inputs=2
  PMSM Controller : eePmsmCurrentController/PMSM Current Controller with Pre-Control  Kp_id=Kdip_sm  Ki_id=Kdii_sm  Kaw_id=0  Kp_iq=Kqip_sm  Ki_iq=Kqii_sm  Kaw_iq=0  Ts=-1  Tsd=0.001  AxisPrio=Q-axis  ActZC=off  ActFF=on  idVect=[-1, 0, 1]  iqVect=[-2000, 0, 2000]  LdMatrix=Ld* ones(3, 3)  LqMatrix=Lq* ones(3, 3)  psimMatrix=psim * ones(3, 3)
  Park Transform : eeTransforms/Park Transform  AxisAlignment=Q-axis  PowerInvariant=off
  Power Controller : Subsystem
  Product : Product
  Scope3 : Scope  NumInputPorts=2
      settings: ActiveDisplayYMinimum=-0.53154558960654574  ActiveDisplayYMaximum=3.2068078785969831  DataLoggingVariableName=ScopeData23
  Selector : Selector  InputPortWidth=3  IndexOptions=Index vector (dialog)  Indices=[1 2]  OutputSizes=1
  Subsystem : Subsystem
  Switch : Switch  Criteria=u2 ~= 0  SaturateOnIntegerOverflow=off  InputSameDT=off
  Unit Delay : UnitDelay  SampleTime=-1
  SM converter control : Outport  VectorParamsAs1DForOutWhenUnconnected=off
  Chopper Control : Outport  Port=2
  wires:
  Product/1 -> Divide/1
  Measurements/1(we) -> PMSM Controller/3
  Unit Delay/1 -> SM converter control/1
  Wind speed/1 -> Power Controller/1(windSpeed)
  Selector/1 -> PMSM Controller/2
  LVRT/1 -> Subsystem/2(LVRT)
  Divide/1 -> Mux1/2
  Constant4/1 -> Switch/3
  Gain1/1 -> Divide1/1
  PMSM Controller/1 -> Mux/1
  Mux1/1 -> Gain2/1
  Power Controller/1(activePowerDemand) -> Product/1
  Divide1/1 -> Unit Delay/1
  Constant2/1 -> Divide/2
  Constant1/1 -> Product/2
  Park Transform/1 -> Selector/1
  iabc_sens/1 -> Measurements/1(iabc_sens)
  Constant/1 -> Mux/2
  Measurements/2(iabc) -> Park Transform/1
  Constant6/1 -> PMSM Controller/5
  Switch/1 -> Divide/3
  Inverse Park Transform/1 -> Gain1/1
  Mux/1 -> Inverse Park Transform/1
  Gain2/1 -> PMSM Controller/1
  Measurements/4(Vdc) -> Subsystem/1(Vdc), Divide1/2
  vdc_sens/1 -> Measurements/4(Vdc_sens)
  Constant5/1 -> PMSM Controller/4
  Subsystem/1(Out1) -> Chopper Control/1
  Gain/1 -> Switch/1, Switch/2
  Constant3/1 -> Mux1/1
  a_sens/1 -> Scope3/2, Measurements/3(th_sens)
  w_sens/1 -> Gain/1, Scope3/1, Measurements/2(w_sens)
  Measurements/3(theta) -> Park Transform/2, Inverse Park Transform/2

== system SimscapeCustomComponents_lib/Microgrid and Renewables/Sources/Wind Plant Integrated/Detailed/Wind Turbine and Converters/Wind Controller/Wind Grid-side Converter Controller ==
  QRef : Inport
  BusElementIn : Inport  Port=2  PortName=VIBus  Element=Vmag
  BusElementIn4 : Inport  Port=2  PortName=VIBus  Element=Vmag
  BusElementIn1 : Inport  Port=2  PortName=VIBus  Element=Iabc
  BusElementIn2 : Inport  Port=2  PortName=VIBus  Element=Vq
  BusElementIn3 : Inport  Port=2  PortName=VIBus  Element=Vd
  BusElementIn5 : Inport  Port=2  PortName=VIBus  Element=Theta
  BusElementIn6 : Inport  Port=2  PortName=VIBus  Element=Theta
  LVRT : Inport  Port=3
  Vdc : Inport  Port=4
  Constant : Constant  Value=Vdc
  Current_controller : Subsystem
  "DC Bus Chopper control " : Subsystem
  DC voltage controller & current reference : Subsystem
  Demux : Demux  Outputs=3
  Inverse Park Transform1 : eeTransforms/Inverse Park Transform  AxisAlignment=Q-axis  PowerInvariant=off
  Park Transform1 : eeTransforms/Park Transform  AxisAlignment=Q-axis  PowerInvariant=off
  Terminator : Terminator
  Unit Delay2 : UnitDelay  SampleTime=Ts
  FRT : Outport
  m_abc : Outport  Port=2
  wires:
  BusElementIn3/1 -> Current_controller/5(Vd)
  BusElementIn1/1 -> Park Transform1/1
  DC voltage controller & current reference/2(iq_ref) -> Current_controller/4(iqref)
  DC voltage controller & current reference/1(id_ref) -> Current_controller/3(id-ref)
  Demux/2 -> Current_controller/2(iq)
  Demux/1 -> Current_controller/1(iWindd)
  Park Transform1/1 -> Demux/1
  BusElementIn2/1 -> Current_controller/6(Vq)
  Inverse Park Transform1/1 -> Unit Delay2/1
  Unit Delay2/1 -> m_abc/1
  Current_controller/1(Refrence_mdq0) -> Inverse Park Transform1/1
  BusElementIn6/1 -> Park Transform1/2
  BusElementIn5/1 -> Inverse Park Transform1/2
  BusElementIn4/1 -> DC voltage controller & current reference/2(Vmag)
  LVRT/1 -> DC voltage controller & current reference/5(lvrt.iq)
  QRef/1 -> DC voltage controller & current reference/1(Q_ref)
  BusElementIn/1 -> "DC Bus Chopper control "/1(In1)
  "DC Bus Chopper control "/1(Out1) -> FRT/1
  Demux/3 -> Terminator/1
  Vdc/1 -> DC voltage controller & current reference/3(Wind_Mpp_vdc)
  Constant/1 -> DC voltage controller & current reference/4(Wind_vdc)

== system SimscapeCustomComponents_lib/Microgrid and Renewables/Sources/Wind Plant Integrated/Detailed/Wind Turbine and Converters/Wind Plant/Back-to-Back Converters ==
  Chopper : Inport
  SM_ref : Inport  Port=2
  Grid_ref : Inport  Port=3
  Average : Subsystem  VariantControl=Average
  Switching : Subsystem  VariantControl=Switching
  In : PMIOPort  Side=Left
  ~ : PMIOPort  Port=2  Side=Right
  Vdc : Outport

== system SimscapeCustomComponents_lib/Microgrid and Renewables/Storage/BESS Integrated/Detailed/BESS Controller/Grid Following/Current_controller ==
  id-ref : Inport
  ipvd : Inport  Port=2
  iqref : Inport  Port=3
  iq : Inport  Port=4
  Vd : Inport  Port=5
  Vq : Inport  Port=6
  Constant4 : Constant  Value=0
  Gain1 : Gain  Gain=2*1*pi*frequency*L/zbase
  Gain2 : Gain  Gain=2*1*pi*frequency*L/zbase
  Mux1 : Mux  Inputs=3
  PID Controller : slpidlib/PID Controller  Controller=PID  Form=Parallel  TimeDomain=Discrete-time  UseExternalTs=off  SampleTime=-1  IntegratorMethod=Forward Euler  FilterMethod=Forward Euler  ControllerParametersSource=internal  P=Kpic  I=Kiic  UseKiTs=off  D=Kd  UseExternalDerivativeSource=off  N=100  UseFilter=on  TunerSelectOption=Transfer Function Based (PID Tuner App)  InitialConditionSource=internal  InitialConditionForIntegrator=0  InitialConditionForFilter=0  DifferentiatorICPrevScaledInput=0  ExternalReset=none  TrackingMode=off  Kt=1  LimitOutput=off  SatLimitsSource=internal  UpperSaturationLimit=inf  LowerSaturationLimit=-inf  LinearizeAsGain=on  AntiWindupMode=none  Kb=1  LimitIntegrator=off  UpperIntegratorSaturationLimit=inf  LowerIntegratorSaturationLimit=-inf  POutMin=[]  POutMax=[]  IOutMin=[]  IOutMax=[]  DOutMin=[]  DOutMax=[]  NOutMin=[]  NOutMax=[]  SumOutMin=[]  SumOutMax=[]  SaturationOutMin=[]  SaturationOutMax=[]  PParamMin=[]  PParamMax=[]  IParamMin=[]  IParamMax=[]  DParamMin=[]  DParamMax=[]  NParamMin=[]  NParamMax=[]  KbParamMin=[]  KbParamMax=[]  KtParamMin=[]  KtParamMax=[]  KbOutMin=[]  KbOutMax=[]  KtOutMin=[]  KtOutMax=[]  IntegratorOutMin=[]  IntegratorOutMax=[]  FilterOutMin=[]  FilterOutMax=[]  SumI1OutMin=[]  SumI1OutMax=[]  SumI2OutMin=[]  SumI2OutMax=[]  SumI3OutMin=[]  SumI3OutMax=[]  SumI4OutMin=[]  SumI4OutMax=[]  SumDOutMin=[]  SumDOutMax=[]  DifferentiatorOutMin=[]  DifferentiatorOutMax=[]  FilterDiffOutCoefMin=[]  FilterDiffOutCoefMax=[]  ReciprocalOutMin=[]  ReciprocalOutMax=[]  SumDenOutMin=[]  SumDenOutMax=[]  SumNumOutMin=[]  SumNumOutMax=[]  DivideOutMin=[]  DivideOutMax=[]  UdiffTsProdOutMin=[]  UdiffTsProdOutMax=[]  NTsProdOutMin=[]  NTsProdOutMax=[]  UintegralTsProdOutMin=[]  UintegralTsProdOutMax=[]  UngainTsProdOutMin=[]  UngainTsProdOutMax=[]  ClampingZeroOutDataTypeStr=Inherit: Inherit via back propagation  ClampingZeroOutMin=[]  ClampingZeroOutMax=[]  FilterDenConstantOutDataTypeStr=Inherit: Inherit via back propagation  FilterDenConstantOutMin=[]  FilterDenConstantOutMax=[]  PCopyOutDataTypeStr=Inherit: Inherit via back propagation  PCopyOutMin=[]  PCopyOutMax=[]  NCopyOutDataTypeStr=Inherit: Inherit via back propagation  NCopyOutMin=[]  NCopyOutMax=[]  IntegratorContinuousStateAttributes=''  IntegratorStateMustResolveToSignalObject=off  IntegratorRTWStateStorageClass=Auto  FilterContinuousStateAttributes=''  FilterStateMustResolveToSignalObject=off  FilterRTWStateStorageClass=Auto  ParallelPVariant=InternalParameters  IdealPVariant=Disabled  IVariant=InternalParameters  DVariant=InternalParameters  IntegratorVariant=Discrete  SatVariant=Disabled  AWVariant=Passthrough  PCopyVariant=Disabled  TRVariant=Disabled  FdbkBlocksVariant=Forward  IdealPFdbkVariant=Disabled  SatFdbkVariant=Disabled  DerivativeFilterVariant=ForwardEulerFilter  NVariant=InternalParameters  NCopyVariant=Disabled  FilterICVariant=InternalICsFilter  IntegratorICVariant=InternalICs  ExternalResetVariant=Disabled  TRSumVariant=Passthrough  SumFdbkVariant=Disabled  SumVariant=Sum_PID  TsampFilterVariant=InternalTs  TsampNgainVariant=Passthrough  TsampIntegralVariant=Disabled_SignalSpec  ExternalSaturationOutDataTypeStr=Inherit: Same as second input  DerivativeSourceVariant=ErrorSignal  PreIntVariant=InternalPreInt
  PID Controller1 : slpidlib/PID Controller  Controller=PID  Form=Parallel  TimeDomain=Discrete-time  UseExternalTs=off  SampleTime=-1  IntegratorMethod=Forward Euler  FilterMethod=Forward Euler  ControllerParametersSource=internal  P=Kpic  I=Kiic  UseKiTs=off  D=Kd  UseExternalDerivativeSource=off  N=100  UseFilter=on  TunerSelectOption=Transfer Function Based (PID Tuner App)  InitialConditionSource=internal  InitialConditionForIntegrator=0  InitialConditionForFilter=0  DifferentiatorICPrevScaledInput=0  ExternalReset=none  TrackingMode=off  Kt=1  LimitOutput=off  SatLimitsSource=internal  UpperSaturationLimit=inf  LowerSaturationLimit=-inf  LinearizeAsGain=on  AntiWindupMode=none  Kb=1  LimitIntegrator=off  UpperIntegratorSaturationLimit=inf  LowerIntegratorSaturationLimit=-inf  POutMin=[]  POutMax=[]  IOutMin=[]  IOutMax=[]  DOutMin=[]  DOutMax=[]  NOutMin=[]  NOutMax=[]  SumOutMin=[]  SumOutMax=[]  SaturationOutMin=[]  SaturationOutMax=[]  PParamMin=[]  PParamMax=[]  IParamMin=[]  IParamMax=[]  DParamMin=[]  DParamMax=[]  NParamMin=[]  NParamMax=[]  KbParamMin=[]  KbParamMax=[]  KtParamMin=[]  KtParamMax=[]  KbOutMin=[]  KbOutMax=[]  KtOutMin=[]  KtOutMax=[]  IntegratorOutMin=[]  IntegratorOutMax=[]  FilterOutMin=[]  FilterOutMax=[]  SumI1OutMin=[]  SumI1OutMax=[]  SumI2OutMin=[]  SumI2OutMax=[]  SumI3OutMin=[]  SumI3OutMax=[]  SumI4OutMin=[]  SumI4OutMax=[]  SumDOutMin=[]  SumDOutMax=[]  DifferentiatorOutMin=[]  DifferentiatorOutMax=[]  FilterDiffOutCoefMin=[]  FilterDiffOutCoefMax=[]  ReciprocalOutMin=[]  ReciprocalOutMax=[]  SumDenOutMin=[]  SumDenOutMax=[]  SumNumOutMin=[]  SumNumOutMax=[]  DivideOutMin=[]  DivideOutMax=[]  UdiffTsProdOutMin=[]  UdiffTsProdOutMax=[]  NTsProdOutMin=[]  NTsProdOutMax=[]  UintegralTsProdOutMin=[]  UintegralTsProdOutMax=[]  UngainTsProdOutMin=[]  UngainTsProdOutMax=[]  ClampingZeroOutDataTypeStr=Inherit: Inherit via back propagation  ClampingZeroOutMin=[]  ClampingZeroOutMax=[]  FilterDenConstantOutDataTypeStr=Inherit: Inherit via back propagation  FilterDenConstantOutMin=[]  FilterDenConstantOutMax=[]  PCopyOutDataTypeStr=Inherit: Inherit via back propagation  PCopyOutMin=[]  PCopyOutMax=[]  NCopyOutDataTypeStr=Inherit: Inherit via back propagation  NCopyOutMin=[]  NCopyOutMax=[]  IntegratorContinuousStateAttributes=''  IntegratorStateMustResolveToSignalObject=off  IntegratorRTWStateStorageClass=Auto  FilterContinuousStateAttributes=''  FilterStateMustResolveToSignalObject=off  FilterRTWStateStorageClass=Auto  ParallelPVariant=InternalParameters  IdealPVariant=Disabled  IVariant=InternalParameters  DVariant=InternalParameters  IntegratorVariant=Discrete  SatVariant=Disabled  AWVariant=Passthrough  PCopyVariant=Disabled  TRVariant=Disabled  FdbkBlocksVariant=Forward  IdealPFdbkVariant=Disabled  SatFdbkVariant=Disabled  DerivativeFilterVariant=ForwardEulerFilter  NVariant=InternalParameters  NCopyVariant=Disabled  FilterICVariant=InternalICsFilter  IntegratorICVariant=InternalICs  ExternalResetVariant=Disabled  TRSumVariant=Passthrough  SumFdbkVariant=Disabled  SumVariant=Sum_PID  TsampFilterVariant=InternalTs  TsampNgainVariant=Passthrough  TsampIntegralVariant=Disabled_SignalSpec  ExternalSaturationOutDataTypeStr=Inherit: Same as second input  DerivativeSourceVariant=ErrorSignal  PreIntVariant=InternalPreInt
  Scope : Scope  NumInputPorts=2
      settings: ActiveDisplayYMinimum=-1  ActiveDisplayYMaximum=1
  Scope1 : Scope  NumInputPorts=2
      settings: ActiveDisplayYMinimum=-1.21282  ActiveDisplayYMaximum=0.9154  DataLoggingVariableName=ScopeData2
  Sum1 : Sum  Inputs=|+-
  Sum3 : Sum  Inputs=|++-
  Sum4 : Sum  Inputs=|+++
  Sum5 : Sum  Inputs=|+-
  mdq0 : Outport
  wires:
  PID Controller/1 -> Sum3/2
  Sum3/1 -> Mux1/1, [Ed]
  Gain2/1 -> Sum3/3
  ipvd/1 -> Scope/2, Gain1/1, Sum1/2
  id-ref/1 -> Scope/1, Sum1/1
  Gain1/1 -> Sum4/3
  Vq/1 -> Sum4/2
  iq/1 -> Scope1/2, Gain2/1, Sum5/2
  Sum1/1 -> PID Controller/1
  Vd/1 -> Sum3/1
  Constant4/1 -> Mux1/3
  Sum5/1 -> PID Controller1/1
  PID Controller1/1 -> Sum4/1
  Sum4/1 -> Mux1/2, [Eq]
  Mux1/1 -> mdq0/1
  iqref/1 -> Scope1/1, Sum5/1

== system SimscapeCustomComponents_lib/Microgrid and Renewables/Storage/BESS Integrated/Detailed/BESS Controller/Grid Following/Reference Current ==
  note: Current Limiters
  note: Avoid division by zero during start
  V_ref : Inport
  V-mag : Inport  Port=2
  del f : Inport  Port=3
  LVRT_iq : Inport  Port=4
  PRef : Inport  Port=5
  QRef : Inport  Port=6
  Constant1 : Constant
  Constant3 : Constant  Value=Imax
  Current limits : Subsystem
  Refernce id generation : Subsystem
  Refernce iq generation : Subsystem
  Switch : Switch  Criteria=u2 ~= 0  SaturateOnIntegerOverflow=off  InputSameDT=off
  Unit Delay1 : UnitDelay  SampleTime=Ts
  Unit Delay3 : UnitDelay  SampleTime=Ts
  id_ref : Outport
  iq_ref : Outport  Port=2
  wires:
  Unit Delay1/1 -> Current limits/2(iqref)
  Current limits/1(iubq) -> Refernce iq generation/1(ubiq)
  Unit Delay3/1 -> Current limits/3(idref)
  Constant3/1 -> Current limits/1(Imax)
  Refernce id generation/1(id_ref) -> id_ref/1, Unit Delay3/1
  del f/1 -> Refernce id generation/2(del f)
  V_ref/1 -> Refernce iq generation/2(V_ref)
  Refernce iq generation/1(iq_ref) -> Unit Delay1/1, iq_ref/1
  LVRT_iq/1 -> Refernce iq generation/4(LVRT_iq)
  V-mag/1 -> Switch/1, Switch/2
  Switch/1 -> Refernce id generation/1(V_mag), Refernce iq generation/3(V_mag)
  Constant1/1 -> Switch/3
  QRef/1 -> Refernce iq generation/5(Q_ref)
  PRef/1 -> Refernce id generation/4(PRef)
  Current limits/2(iubd) -> Refernce id generation/3(ubid)

== system SimscapeCustomComponents_lib/Microgrid and Renewables/Storage/BESS Integrated/Detailed/BESS Controller/Grid Forming/Current Limiting ==
  In Bus Element : Inport  PortName=measure  Element=Igd
  In Bus Element1 : Inport  PortName=measure  Element=Igq
  In Bus Element2 : Inport  Port=2  PortName=reactiveControl  Element=Vmd
  In Bus Element4 : Inport  Port=2  PortName=reactiveControl  Element=Vmq
  CurrentLimitingMethod : Subsystem  Variant=on  VariantControlMode=label  VariantControl=Choice  LabelModeActiveChoice=ctSat
  Scope : Scope  NumInputPorts=2
  Subtract : Sum  Inputs=+-
  Subtract1 : Sum  Inputs=-+
  Out Bus Element : Outport  PortName=currentLimiting  Element=Vmd
  Out Bus Element1 : Outport  PortName=currentLimiting  Element=Vmq
  Out Bus Element2 : Outport  PortName=currentLimiting  Element=Idmax
  Out Bus Element3 : Outport  PortName=currentLimiting  Element=Iqmax
  wires:
  In Bus Element2/1 -> Subtract/1
  In Bus Element1/1 -> CurrentLimitingMethod/2(Igq)
  In Bus Element4/1 -> Subtract1/2
  Subtract/1 -> Scope/1, Out Bus Element/1
  Subtract1/1 -> Scope/2, Out Bus Element1/1
  CurrentLimitingMethod/4(Iqmax) -> Out Bus Element3/1
  In Bus Element/1 -> CurrentLimitingMethod/1(Igd)  "Q"
  CurrentLimitingMethod/3(Idmax) -> Out Bus Element2/1
  CurrentLimitingMethod/1(delVd) -> Subtract/2
  CurrentLimitingMethod/2(delVq) -> Subtract1/1
